simulink model "BouncingMass_Model"  (R2023b)
settings: Solver=VariableStepAuto  StartTime=0.0  StopTime=10.0  RelTol=1e-3
model workspace (MAT data in the model file):
  c = Simulink.Parameter
  c.Value = 5
  c.DataType = 'auto'
  c.Complexity = 'real'
  c.Dimensions = [1 1]
  g = Simulink.Parameter
  g.Value = 9.81
  g.DataType = 'auto'
  g.Complexity = 'real'
  g.Dimensions = [1 1]
  k = Simulink.Parameter
  k.Value = 2000
  k.DataType = 'auto'
  k.Complexity = 'real'
  k.Dimensions = [1 1]
  m = Simulink.Parameter
  m.Value = 5
  m.DataType = 'auto'
  m.Complexity = 'real'
  m.Dimensions = [1 1]
values from neighbouring files (symbols this model uses):
  g = 9.81    [BumpBump.m]    (also in quarter_car_model_ss.m; runBumpBump.m)
  k = k*mR    [BumpBump.m]    (also in LongitudinalPower.m = 4800; runBumpBump.m = 10509.0590551)
  m = m*.4535    (= 47.6175)    [runBumpBump.m]
libraries: simulink x2
settings Model: Creator=arnav  LastModifiedBy=arnav

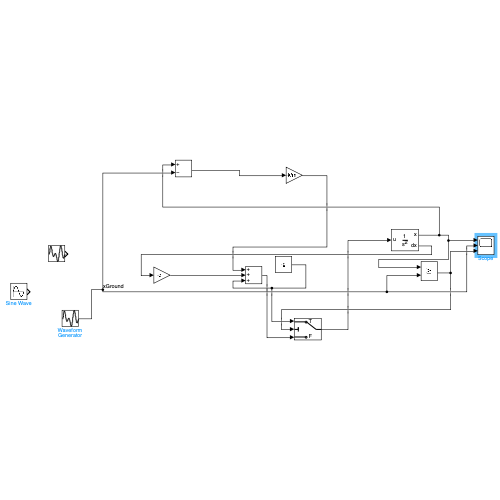
[thumbnail: Simulink's stored preview of the top-level diagram]
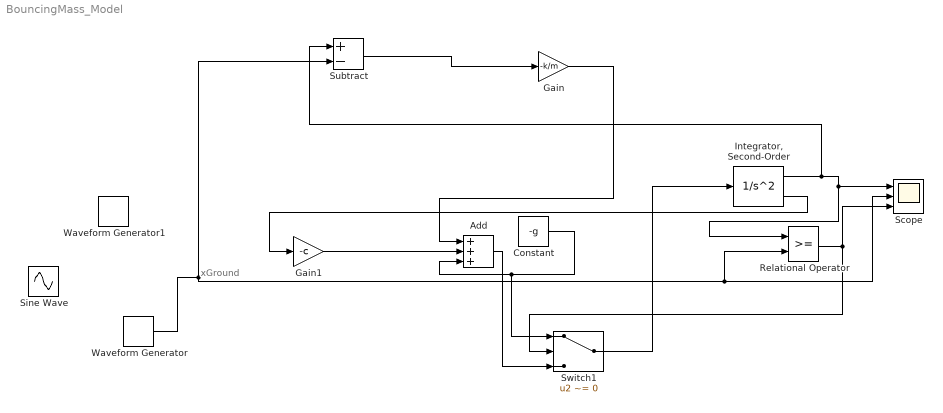
== system BouncingMass_Model ==
  note: xGround
  Add : Sum  Inputs=+++
  Constant : Constant  Value=-g
  Gain : Gain  Gain=-k/m
  Gain1 : Gain  Gain=-c
  "Integrator, Second-Order" : SecondOrderIntegrator
  Relational Operator : RelationalOperator  OutDataTypeStr=boolean  RndMeth=Simplest  InputSameDT=off
  Scope : Scope  NumInputPorts=3
  Sine Wave : Sin  Amplitude=-1  Phase=-pi/2  SampleTime=0
  Subtract : Sum  Inputs=+-
  Switch1 : Switch  Criteria=u2 ~= 0  SaturateOnIntegerOverflow=off  InputSameDT=off
  Waveform Generator : simulink/Sources/Waveform Generator  OutMin=[]  OutMax=[]  OutDataTypeStr=double  SelectedSignal=1  Signals=step('StepTime',5,'InitialValue',0,'FinalValue',-3)  BlockNames=MultiportSwitch_9a5769d9e4dc4c3  SampleTime=0.1
  Waveform Generator1 : simulink/Sources/Waveform Generator  OutMin=[]  OutMax=[]  OutDataTypeStr=double  SelectedSignal=1  BlockNames=MultiportSwitch_e3df3653d217406  SampleTime=0.1
  wires:
  "Integrator, Second-Order"/1 -> Subtract/1, Scope/1, Relational Operator/1
  Waveform Generator/1 -> Relational Operator/2, Scope/2, Subtract/2
  Subtract/1 -> Gain/1
  "Integrator, Second-Order"/2 -> Gain1/1
  Gain/1 -> Add/1
  Gain1/1 -> Add/2
  Relational Operator/1 -> Scope/3, Switch1/2
  Constant/1 -> Add/3, Switch1/1
  Add/1 -> Switch1/3
  Switch1/1 -> "Integrator, Second-Order"/1
